simulink model "Banco_Seguridad_Stateflow"  (R2025b)
settings: Solver=FixedStepDiscrete  StartTime=0.0  StopTime=0.6  FixedStep=0.02  RelTol=1e-3
InitFcn:
  | T_s0=0.02;
settings Model: Creator=meesc  LastModifiedBy=meesc
settings DataIOCC: SaveOutput=off  SignalLogging=off

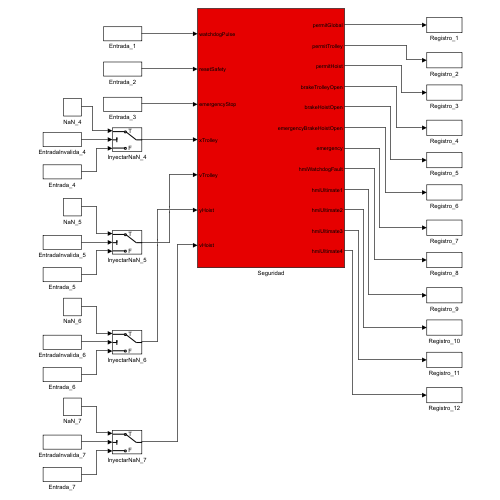
[thumbnail: Simulink's stored preview of the top-level diagram]
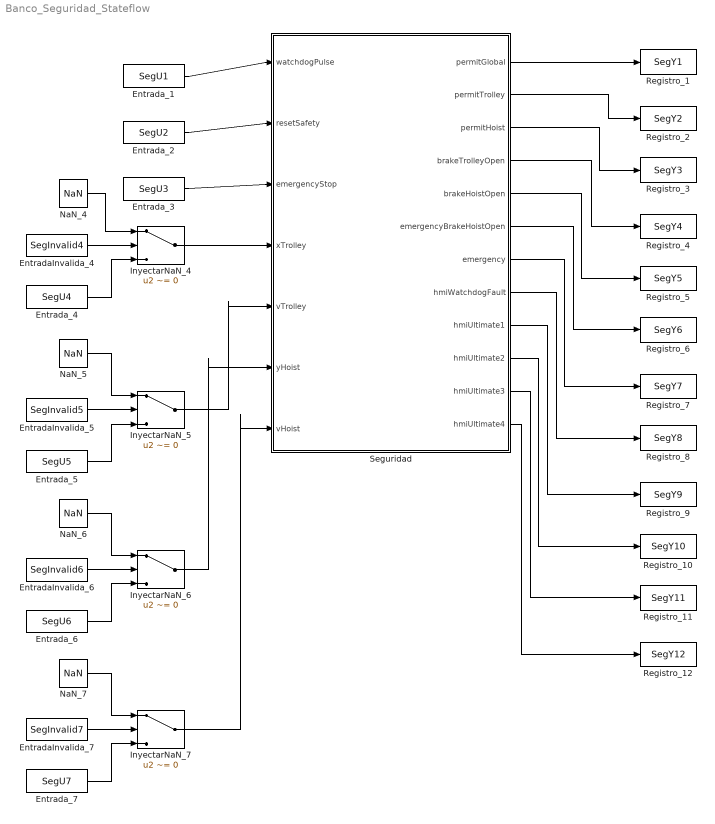
== system Banco_Seguridad_Stateflow ==
  EntradaInvalida_4 : FromWorkspace  VariableName=SegInvalid4  Interpolate=off  OutputAfterFinalValue=Holding final value
  EntradaInvalida_5 : FromWorkspace  VariableName=SegInvalid5  Interpolate=off  OutputAfterFinalValue=Holding final value
  EntradaInvalida_6 : FromWorkspace  VariableName=SegInvalid6  Interpolate=off  OutputAfterFinalValue=Holding final value
  EntradaInvalida_7 : FromWorkspace  VariableName=SegInvalid7  Interpolate=off  OutputAfterFinalValue=Holding final value
  Entrada_1 : FromWorkspace  VariableName=SegU1  Interpolate=off  OutputAfterFinalValue=Holding final value
  Entrada_2 : FromWorkspace  VariableName=SegU2  Interpolate=off  OutputAfterFinalValue=Holding final value
  Entrada_3 : FromWorkspace  VariableName=SegU3  Interpolate=off  OutputAfterFinalValue=Holding final value
  Entrada_4 : FromWorkspace  VariableName=SegU4  Interpolate=off  OutputAfterFinalValue=Holding final value
  Entrada_5 : FromWorkspace  VariableName=SegU5  Interpolate=off  OutputAfterFinalValue=Holding final value
  Entrada_6 : FromWorkspace  VariableName=SegU6  Interpolate=off  OutputAfterFinalValue=Holding final value
  Entrada_7 : FromWorkspace  VariableName=SegU7  Interpolate=off  OutputAfterFinalValue=Holding final value
  InyectarNaN_{4..7} (4 alike) : Switch  Criteria=u2 ~= 0  SaturateOnIntegerOverflow=off  InputSameDT=off
  NaN_{4..7} (4 alike) : Constant  Value=NaN
  Registro_1 : ToWorkspace  VariableName=SegY1  SaveFormat=Timeseries  SampleTime=-1
  Registro_10 : ToWorkspace  VariableName=SegY10  SaveFormat=Timeseries  SampleTime=-1
  Registro_11 : ToWorkspace  VariableName=SegY11  SaveFormat=Timeseries  SampleTime=-1
  Registro_12 : ToWorkspace  VariableName=SegY12  SaveFormat=Timeseries  SampleTime=-1
  Registro_2 : ToWorkspace  VariableName=SegY2  SaveFormat=Timeseries  SampleTime=-1
  Registro_3 : ToWorkspace  VariableName=SegY3  SaveFormat=Timeseries  SampleTime=-1
  Registro_4 : ToWorkspace  VariableName=SegY4  SaveFormat=Timeseries  SampleTime=-1
  Registro_5 : ToWorkspace  VariableName=SegY5  SaveFormat=Timeseries  SampleTime=-1
  Registro_6 : ToWorkspace  VariableName=SegY6  SaveFormat=Timeseries  SampleTime=-1
  Registro_7 : ToWorkspace  VariableName=SegY7  SaveFormat=Timeseries  SampleTime=-1
  Registro_8 : ToWorkspace  VariableName=SegY8  SaveFormat=Timeseries  SampleTime=-1
  Registro_9 : ToWorkspace  VariableName=SegY9  SaveFormat=Timeseries  SampleTime=-1
  Seguridad : Subsystem
  wires:
  Entrada_1/1 -> Seguridad/1(watchdogPulse)
  NaN_4/1 -> InyectarNaN_4/1
  EntradaInvalida_4/1 -> InyectarNaN_4/2
  Entrada_4/1 -> InyectarNaN_4/3
  EntradaInvalida_6/1 -> InyectarNaN_6/2
  NaN_5/1 -> InyectarNaN_5/1
  NaN_6/1 -> InyectarNaN_6/1
  EntradaInvalida_5/1 -> InyectarNaN_5/2
  InyectarNaN_6/1 -> Seguridad/6(yHoist)
  Entrada_5/1 -> InyectarNaN_5/3
  Entrada_6/1 -> InyectarNaN_6/3
  Entrada_2/1 -> Seguridad/2(resetSafety)
  NaN_7/1 -> InyectarNaN_7/1
  EntradaInvalida_7/1 -> InyectarNaN_7/2
  Entrada_7/1 -> InyectarNaN_7/3
  Entrada_3/1 -> Seguridad/3(emergencyStop)
  Seguridad/7(emergency) -> Registro_7/1
  InyectarNaN_4/1 -> Seguridad/4(xTrolley)
  Seguridad/9(hmiUltimate1) -> Registro_9/1
  InyectarNaN_5/1 -> Seguridad/5(vTrolley)
  InyectarNaN_7/1 -> Seguridad/7(vHoist)
  Seguridad/1(permitGlobal) -> Registro_1/1
  Seguridad/2(permitTrolley) -> Registro_2/1
  Seguridad/3(permitHoist) -> Registro_3/1
  Seguridad/4(brakeTrolleyOpen) -> Registro_4/1
  Seguridad/5(brakeHoistOpen) -> Registro_5/1
  Seguridad/6(emergencyBrakeHoistOpen) -> Registro_6/1
  Seguridad/8(hmiWatchdogFault) -> Registro_8/1
  Seguridad/10(hmiUltimate2) -> Registro_10/1
  Seguridad/11(hmiUltimate3) -> Registro_11/1
  Seguridad/12(hmiUltimate4) -> Registro_12/1

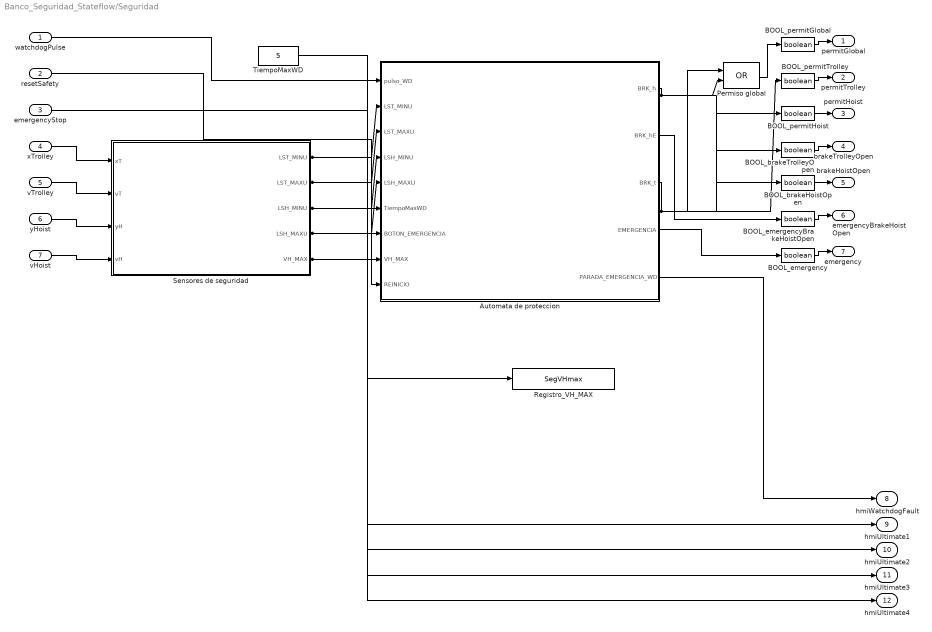
== system Banco_Seguridad_Stateflow/Seguridad ==
  watchdogPulse : Inport
  resetSafety : Inport  Port=2
  emergencyStop : Inport  Port=3
  xTrolley : Inport  Port=4
  vTrolley : Inport  Port=5
  yHoist : Inport  Port=6
  vHoist : Inport  Port=7
  Automata de proteccion : Stateflow chart  TreatAsAtomicUnit=on
      settings: PortSchema="{\"entries\":[{\"content\":{\"sides\":[{\"content\":{\"connectorIds\":[\"In1\",\"In3\",\"In4\",\"In5\",\"In6\",\"In7\",\"In8\",\"In9\",\"In2\"]},\"type\":\"ConnectorPlacement.EquallySpacedRectSide\",\"uuid\":\"cd0792a4-97ef-4c80-9019-d76753964359\"},{\"content\":{\"connectorIds\":[\"Out1\",\"Out2\",\"Out3\",\"Out4\",\"Out5\"],\"side\":\"RIGHT\"},\"type\":\"ConnectorPlacement.EquallySpacedRectSide\",\"uuid\":\"2986dd5d-2111-4155-8673-f52c044c46ad\"},{\"content\":{\"side\":\"TOP\"},\"type\":\"ConnectorPlacement.EquallySpacedRectSide\",\"uuid\":\"d52e82c5-c118-49d3-899a-ea936e299c34\"}]},\"type\":\"ConnectorPlacement.EquallySpacedConnector\",\"uuid\":\"580a1a82-6a30-4652-9187-78ca47e5d1d9\"}],\"packageUris\":[\"http://schema.mathworks.com/mf0/Connector/R2020b\"],\"version\":\"1.0\"}"
  BOOL_brakeHoistOpen : DataTypeConversion  OutDataTypeStr=boolean  SaturateOnIntegerOverflow=off  RndMeth=Floor
  BOOL_brakeTrolleyOpen : DataTypeConversion  OutDataTypeStr=boolean  SaturateOnIntegerOverflow=off  RndMeth=Floor
  BOOL_emergency : DataTypeConversion  OutDataTypeStr=boolean  SaturateOnIntegerOverflow=off  RndMeth=Floor
  BOOL_emergencyBrakeHoistOpen : DataTypeConversion  OutDataTypeStr=boolean  SaturateOnIntegerOverflow=off  RndMeth=Floor
  BOOL_permitGlobal : DataTypeConversion  OutDataTypeStr=boolean  SaturateOnIntegerOverflow=off  RndMeth=Floor
  BOOL_permitHoist : DataTypeConversion  OutDataTypeStr=boolean  SaturateOnIntegerOverflow=off  RndMeth=Floor
  BOOL_permitTrolley : DataTypeConversion  OutDataTypeStr=boolean  SaturateOnIntegerOverflow=off  RndMeth=Floor
  Permiso global : Logic  Operator=OR  AllPortsSameDT=off  OutDataTypeStr=boolean
  Registro_VH_MAX : ToWorkspace  VariableName=SegVHmax  SaveFormat=Timeseries  SampleTime=-1
  Sensores de seguridad : MATLAB Function  TreatAsAtomicUnit=on
  TiempoMaxWD : Constant  Value=5  OutDataTypeStr=double
  permitGlobal : Outport
  permitTrolley : Outport  Port=2
  permitHoist : Outport  Port=3
  brakeTrolleyOpen : Outport  Port=4
  brakeHoistOpen : Outport  Port=5
  emergencyBrakeHoistOpen : Outport  Port=6
  emergency : Outport  Port=7
  hmiWatchdogFault : Outport  Port=8
  hmiUltimate1 : Outport  Port=9
  hmiUltimate2 : Outport  Port=10
  hmiUltimate3 : Outport  Port=11
  hmiUltimate4 : Outport  Port=12
  wires:
  Automata de proteccion/5(PARADA_EMERGENCIA_WD) -> hmiWatchdogFault/1
  BOOL_emergency/1 -> emergency/1
  Automata de proteccion/4(EMERGENCIA) -> BOOL_emergency/1
  BOOL_emergencyBrakeHoistOpen/1 -> emergencyBrakeHoistOpen/1
  Automata de proteccion/2(BRK_hE) -> BOOL_emergencyBrakeHoistOpen/1
  BOOL_brakeHoistOpen/1 -> brakeHoistOpen/1
  BOOL_brakeTrolleyOpen/1 -> brakeTrolleyOpen/1
  BOOL_permitHoist/1 -> permitHoist/1
  BOOL_permitTrolley/1 -> permitTrolley/1
  BOOL_permitGlobal/1 -> permitGlobal/1
  Permiso global/1 -> BOOL_permitGlobal/1
  Automata de proteccion/1(BRK_h) -> BOOL_brakeHoistOpen/1, BOOL_permitHoist/1, Permiso global/2
  Automata de proteccion/3(BRK_t) -> BOOL_brakeTrolleyOpen/1, BOOL_permitTrolley/1, Permiso global/1
  Sensores de seguridad/5(VH_MAX) -> Automata de proteccion/9(VH_MAX), Registro_VH_MAX/1
  emergencyStop/1 -> Automata de proteccion/8(BOTON_EMERGENCIA)
  TiempoMaxWD/1 -> Automata de proteccion/7(TiempoMaxWD)
  Sensores de seguridad/4(LSH_MAXU) -> hmiUltimate4/1, Automata de proteccion/6(LSH_MAXU)
  Sensores de seguridad/3(LSH_MINU) -> hmiUltimate3/1, Automata de proteccion/5(LSH_MINU)
  Sensores de seguridad/2(LST_MAXU) -> hmiUltimate2/1, Automata de proteccion/4(LST_MAXU)
  Sensores de seguridad/1(LST_MINU) -> hmiUltimate1/1, Automata de proteccion/3(LST_MINU)
  resetSafety/1 -> Automata de proteccion/2(REINICIO)
  watchdogPulse/1 -> Automata de proteccion/1(pulso_WD)
  vHoist/1 -> Sensores de seguridad/4(vH)
  yHoist/1 -> Sensores de seguridad/3(yH)
  vTrolley/1 -> Sensores de seguridad/2(vT)
  xTrolley/1 -> Sensores de seguridad/1(xT)

== stateflow chart Banco_Seguridad_Stateflow/Seguridad/Automata de proteccion ==
  settings: updateMethod=DISCRETE  sampleTime=T_s0
  state SALTOS_EMERGENCIAS [parallel]
    settings: executionOrder=1
    state FUNCIONAMIENTO_NORMAL
      entry:
      EMERGENCIA=false;
      BRK_t=true;
      BRK_h=true;
      BRK_hE=true;
    state EMERGENCIA_IZAJE
      entry:
      EMERGENCIA=true;
      BRK_t=true;
      BRK_h=false;
      BRK_hE=false;
    state EMERGENCIA_CARRO
      entry:
      EMERGENCIA=true;
      BRK_t=false;
      BRK_h=true;
      BRK_hE=true;
    state EMERGENCIA_TOTAL
      entry:
      EMERGENCIA=true;
      BRK_t=false;
      BRK_h=false;
      BRK_hE=false;
    (default) -> SALTOS_EMERGENCIAS.FUNCIONAMIENTO_NORMAL
    SALTOS_EMERGENCIAS.FUNCIONAMIENTO_NORMAL -> EMERGENCIA_CARRO [order 3] : [hasChangedTo(LST_MAXU,1) || hasChangedTo(LST_MINU,1)]
    SALTOS_EMERGENCIAS.FUNCIONAMIENTO_NORMAL -> EMERGENCIA_IZAJE [order 2] : [hasChangedTo(LSH_MAXU,1) || hasChangedTo(LSH_MINU,1) || hasChangedTo(VH_MAX,1)]
    EMERGENCIA_CARRO -> SALTOS_EMERGENCIAS.FUNCIONAMIENTO_NORMAL [order 2] : [~BOTON_EMERGENCIA && ~LST_MAXU && ~LST_MINU && hasChangedTo(REINICIO,1)]
    EMERGENCIA_IZAJE -> SALTOS_EMERGENCIAS.FUNCIONAMIENTO_NORMAL [order 2] : [~BOTON_EMERGENCIA && ~LSH_MAXU && ~LSH_MINU && ~VH_MAX && hasChangedTo(REINICIO,1)]
    SALTOS_EMERGENCIAS.FUNCIONAMIENTO_NORMAL -> EMERGENCIA_TOTAL [order 1] : [BOTON_EMERGENCIA || PARADA_EMERGENCIA_WD]
    EMERGENCIA_TOTAL -> SALTOS_EMERGENCIAS.FUNCIONAMIENTO_NORMAL : [~BOTON_EMERGENCIA && ~PARADA_EMERGENCIA_WD && ~LST_MAXU && ~LST_MINU && ~LSH_MAXU && ~LSH_MINU && ~VH_MAX && hasChangedTo(REINICIO,1)]
    EMERGENCIA_CARRO -> EMERGENCIA_TOTAL [order 1] : [hasChangedTo(LSH_MAXU,1) || hasChangedTo(LSH_MINU,1) || hasChangedTo(VH_MAX,1) || BOTON_EMERGENCIA || PARADA_EMERGENCIA_WD]
    EMERGENCIA_IZAJE -> EMERGENCIA_TOTAL [order 1] : [hasChangedTo(LST_MAXU,1) || hasChangedTo(LST_MINU,1) || BOTON_EMERGENCIA || PARADA_EMERGENCIA_WD]
  state WATCHDOG [parallel]
    settings: executionOrder=2
    state FUNCIONAMIENTO_NORMAL
      entry:
      PARADA_EMERGENCIA_WD=false;
    state FALLO_WD
      entry:
      PARADA_EMERGENCIA_WD=true;
    (default) -> WATCHDOG.FUNCIONAMIENTO_NORMAL
    FALLO_WD -> WATCHDOG.FUNCIONAMIENTO_NORMAL : [hasChangedTo(REINICIO,1)]
    WATCHDOG.FUNCIONAMIENTO_NORMAL -> WATCHDOG.FUNCIONAMIENTO_NORMAL [order 2] : [hasChanged(pulso_WD)]
    WATCHDOG.FUNCIONAMIENTO_NORMAL -> FALLO_WD [order 1] : [after(TiempoMaxWD, sec)]
  data: pulso_WD input boolean; REINICIO input boolean; BRK_h output boolean; BRK_hE output boolean; BRK_t output boolean; EMERGENCIA output boolean; LST_MINU input boolean; LST_MAXU input boolean; LSH_MINU input boolean; LSH_MAXU input boolean; TiempoMaxWD input double =10; BOTON_EMERGENCIA input boolean; VH_MAX input boolean; PARADA_EMERGENCIA_WD output boolean

== matlab function Banco_Seguridad_Stateflow/Seguridad/Sensores de seguridad ==
  data: xT input; LST_MINU output; vT input; yH input; vH input; LST_MAXU output; LSH_MINU output; LSH_MAXU output; VH_MAX output
function [LST_MINU,LST_MAXU,LSH_MINU,LSH_MAXU,VH_MAX] = detectar(xT,vT,yH,vH)
%#codegen
LST_MINU = (xT <= -30.5) || (vT <= -4.6);
LST_MAXU = (xT >=  50.5) || (vT >=  4.6);
LSH_MINU = yH <= -20.5;
LSH_MAXU = yH >=  40.5;
VH_MAX = abs(vH) >= 3.45;
end
